simulink model "Electrical_System_2018b_obfs"  (R2019b)
settings: Solver=VariableStepAuto  StartTime=0.0  StopTime=5  RelTol=1e-3  AbsTol=1e-3  EnableMultiTasking=on
InitFcn:
  | Steady_State_Initialisation;
StopFcn:
  | %sscexplore(simlog);
  | %Logging
undefined symbols (not defined in the file): abrlhklxvp, aexgmhuedq, afmfmjnutg, afpphrjpnc, ahuxbyvruc, alarvljztt, amxnyqmnuw, aodrlwvqie, aolhmuplyq, aqpmguuqkg, auesgwirzl, aurophlnng, awamelrhru, ayfhvxflxn, azxkacuhqc, babszerikg, bawhdqanwq, bevoqecvei, bltjvqbchx, bmqsuewujl, bsmyqjfgnf, btvjbsmnve, bywgxqeadw, bziaduxaer, bzmcmdqocb, bzsvyvetat, ccsjnrbsih, cdvenygxwh, cedkrnslhx, cjheorclzs, cjrdshrtqx, ckhavyhcza, ckxewznhlz, cmrcgyiplk, conenicnws, cqkejbgjnn, csfnuwymhe, cunupkhwbh, cwzfvzuxxh, dcadmadufn, dcfponivnv, ddtrqjrhjn, dfhoxvkqas, dfrhtcwpne, dfvomcagjv, djijwylxea, dnmeqksrrm, dnzewbdkaa, dsqcykyxav, dtswwlttmm, ecumpidjtv, edegaywrct, ejjjsmnejc, eknqnehjdz, emvdetzouf, esxbqkbahr, etnkkbreiq, eunoiiiirw, ewewcuedir, fatkfxdhtc ... (+386)
libraries: fl_lib x802, ee_lib x362, fl_ps_legacy_lib x160, nesl_utility x85
(part 12 of 26)

== system Electrical_System_2018b_obfs/Redacted_1221/Redacted_7996/Redacted_1/Redacted_4377/Redacted_6082/Redacted_6448 ==
  Redacted_2500 : ee_lib/Semiconductors & Converters/Diode  ModelType=efectnzfzk  Vf=jxmepmeowj V  Ron=qgxsnpyvap Ohm  Goff=yoppabgzkl S  prmExp=ubpcccmurz  I12=remshksgqe A  V12=lfyuowwnsp V  IS=kniawzssyt A  ec=shjfprvpho  I1=bqvkznozbx A  V1=kanhzjgbwy V  RS=xqskwtorcu Ohm  Tmeas=wkndwwjeju degC  N_series=oemgleyaog  N_parallel=rmwesacawc  Rz=uupgbnboph Ohm  BV=jmlshjudem V  C_param=ejznuqydbf  CJ=jnyvftnijl pF  CJ0=eocfcshsjc pF  VJ=rcqumjutus V  Mgrad=bpwyttzsav  Vvec=xmbkulzqwe V  Cvec=eqgbafiqja pF  FC=fzcbcscgmr  Q_param=hevnohlimn  iRM=fkisxhzojn A  iF=aecufenajy A  didt=wqayegsgya A/us  trr_factor=tyozkzrsye  trr=byygrqxzxs ns  Qrr=ecsprgxdxa s*uA  TT=estselsvjb ns  tau=lnvjuifvwe ns  T_param=jrnxklcvyp  IS_T2=pegzeyggnh A  I1_T2=dfmjfojaum A  V1_T2=dkkcmajvzi V  Tmeas2=mhkasfkmys degC  EG_param=agwssckltu  EG=rfaarmrbja eV  XTI_param=uxzupvrblg  XTI=ospysejegc  dBVdT=tootsfdmyr V/K  Tdevice=kzpnsiiwfr degC  i_specify=off  i_priority=None  i=eihvzvfrzd A  i_nominal_specify=off  i_nominal_unit=A  i_nominal_value=qmmhrurogd  v_specify=off  v_priority=None  v=hizlbruxfz V  v_nominal_specify=off  v_nominal_unit=V  v_nominal_value=ycpyizpqai  i_capacitor_specify=off  i_capacitor_priority=None  i_capacitor=zppifvcjba A  i_capacitor_nominal_specify=off  i_capacitor_nominal_unit=A  i_capacitor_nominal_value=fpmjfabdfd  v_capacitor_specify=off  v_capacitor_priority=None  v_capacitor=stollmyrll V  v_capacitor_nominal_specify=off  v_capacitor_nominal_unit=V  v_capacitor_nominal_value=kndonlhkoo  power_dissipated_specify=off  power_dissipated_priority=None  power_dissipated=btdavdcdiv W  power_dissipated_nominal_specify=off  power_dissipated_nominal_unit=W  power_dissipated_nominal_value=tkklgbzblp  thermal_network_parameterization=bljrklmcju  Rth=xhsqylwmob K/W  Rth_Foster=optpcutsoi K/W  thermal_mass_parameterization=ugcqtdtype  thermal_mass=jsyutsyost J/K  thermal_mass_Foster=twrmylwkjc J/K  thermal_time_constant=xnykkposzd s  thermal_time_constant_Foster=foiqukjmop s  thermal_mass_initial_temperatures=upiyseqegs degC
      settings: SourceProductName=Simscape Electrical  InternalSimscapePortConfiguration="{\"Bottom\":[],\"Left\":[{\"id\":\"p\",\"label\":\"\",\"type\":\"foundation.electrical.electrical\"},{\"id\":\"H\",\"label\":\"H\",\"type\":\"foundation.thermal.thermal\"}],\"Right\":[{\"id\":\"n\",\"label\":\"\",\"type\":\"foundation.electrical.electrical\"}],\"Top\":[]}"
  Redacted_359 : ee_lib/Semiconductors & Converters/Diode  ModelType=scvaiquffk  Vf=gurupglfta V  Ron=ftlaqddzvo Ohm  Goff=sbgfdffxay S  prmExp=ukcnmjtiae  I12=grbxogokac A  V12=wmzyrlvpsn V  IS=leyegtjcol A  ec=lwvjfwcdkf  I1=dljtokvayx A  V1=irawojoicp V  RS=axoqkcbxfn Ohm  Tmeas=aargryzkwo degC  N_series=kaksezvljy  N_parallel=xdnjyjftou  Rz=rcunxliptk Ohm  BV=hrrjansjso V  C_param=gklskhmoru  CJ=imyuobqtwk pF  CJ0=ewdqrpecjy pF  VJ=wfjksexohd V  Mgrad=jgqtcmmwqv  Vvec=aguvzvrglj V  Cvec=zssvjevjde pF  FC=oeclxcixjt  Q_param=xrpxrrdafl  iRM=bcqzohazjt A  iF=crytmcfhbt A  didt=sirllclhmt A/us  trr_factor=ziidcweruu  trr=wxebnnxvyt ns  Qrr=ausdiytbgo s*uA  TT=naewcxqzgl ns  tau=ctbkxtppav ns  T_param=kyxkskcyft  IS_T2=nshgzahsri A  I1_T2=xuvyuqjsme A  V1_T2=oltorpmvrx V  Tmeas2=gktjbxgqtx degC  EG_param=iwktfixgrg  EG=teimjuixxi eV  XTI_param=shpugjdkdk  XTI=yrdjcsecbk  dBVdT=volhbyrkkf V/K  Tdevice=ofrafibacf degC  i_specify=off  i_priority=None  i=qtezljymoi A  i_nominal_specify=off  i_nominal_unit=A  i_nominal_value=yxnhkqaqti  v_specify=off  v_priority=None  v=kbwxruyprv V  v_nominal_specify=off  v_nominal_unit=V  v_nominal_value=igljubvsuu  i_capacitor_specify=off  i_capacitor_priority=None  i_capacitor=mlyqgxdfvw A  i_capacitor_nominal_specify=off  i_capacitor_nominal_unit=A  i_capacitor_nominal_value=ujbiigzksz  v_capacitor_specify=off  v_capacitor_priority=None  v_capacitor=cojyhmmzxj V  v_capacitor_nominal_specify=off  v_capacitor_nominal_unit=V  v_capacitor_nominal_value=wujzjvntdo  power_dissipated_specify=off  power_dissipated_priority=None  power_dissipated=yxytktehoc W  power_dissipated_nominal_specify=off  power_dissipated_nominal_unit=W  power_dissipated_nominal_value=pjafufeysq  thermal_network_parameterization=tftjmfuyfl  Rth=qburaojkwt K/W  Rth_Foster=jtrsywfksp K/W  thermal_mass_parameterization=mpaelmbuic  thermal_mass=qbntcmqzdf J/K  thermal_mass_Foster=iddtfueyvm J/K  thermal_time_constant=ewlbqfzhqf s  thermal_time_constant_Foster=ircpsmtrsx s  thermal_mass_initial_temperatures=xmifunpacs degC
      settings: SourceProductName=Simscape Electrical  InternalSimscapePortConfiguration="{\"Bottom\":[],\"Left\":[{\"id\":\"p\",\"label\":\"\",\"type\":\"foundation.electrical.electrical\"},{\"id\":\"H\",\"label\":\"H\",\"type\":\"foundation.thermal.thermal\"}],\"Right\":[{\"id\":\"n\",\"label\":\"\",\"type\":\"foundation.electrical.electrical\"}],\"Top\":[]}"
  Redacted_4119 : fl_lib/Electrical/Electrical Elements/Switch  R_closed=nvzhbxdgzi Ohm  G_open=jocuywfdlu 1/Ohm  Threshold=ycxpvyjhxx  i_specify=off  i_priority=None  i=wyjfxhkfvg A  i_nominal_specify=off  i_nominal_unit=A  i_nominal_value=qhiybsolgq  v_specify=off  v_priority=None  v=qhliplaqbe V  v_nominal_specify=off  v_nominal_unit=V  v_nominal_value=dflzoctfhv
      settings: SourceProductName=Simscape
  Redacted_7045 : ee_lib/Passive/Thermal/Thermal Resistor  R=znufdvpgrp K/W  T_specify=off  T_priority=None  T=gjhwzpgvuf K  T_nominal_specify=off  T_nominal_unit=K  T_nominal_value=wamkuaqotp  Q_specify=off  Q_priority=None  Q=iffnecxdnj W  Q_nominal_specify=off  Q_nominal_unit=W  Q_nominal_value=vfrfuelbtd
      settings: SourceProductName=Simscape Electrical  SourceProductBaseCode=PS  InternalSimscapePortConfiguration="{\"Bottom\":[],\"Left\":[{\"id\":\"A\",\"label\":\"A\",\"type\":\"foundation.thermal.thermal\"}],\"Right\":[{\"id\":\"B\",\"label\":\"B\",\"type\":\"foundation.thermal.thermal\"}],\"Top\":[]}"
  Redacted_7113 : fl_lib/Electrical/Electrical Elements/Switch  R_closed=xpgttbnlcv Ohm  G_open=qgroafvezw 1/Ohm  Threshold=emvdetzouf  i_specify=off  i_priority=None  i=kqcxlhjixi A  i_nominal_specify=off  i_nominal_unit=A  i_nominal_value=serpbanljy  v_specify=off  v_priority=None  v=tquhywvxiq V  v_nominal_specify=off  v_nominal_unit=V  v_nominal_value=hqozyjemvy
      settings: SourceProductName=Simscape
  Redacted_7754 : ee_lib/Passive/Thermal/Thermal Resistor  R=pifghqliop K/W  T_specify=off  T_priority=None  T=liaimvkskv K  T_nominal_specify=off  T_nominal_unit=K  T_nominal_value=plbwxvjplh  Q_specify=off  Q_priority=None  Q=nitcggggrk W  Q_nominal_specify=off  Q_nominal_unit=W  Q_nominal_value=cufaoxszsm
      settings: SourceProductName=Simscape Electrical  SourceProductBaseCode=PS  InternalSimscapePortConfiguration="{\"Bottom\":[],\"Left\":[{\"id\":\"A\",\"label\":\"A\",\"type\":\"foundation.thermal.thermal\"}],\"Right\":[{\"id\":\"B\",\"label\":\"B\",\"type\":\"foundation.thermal.thermal\"}],\"Top\":[]}"
  Redacted_8069 : ee_lib/Passive/Thermal/Thermal Resistor  R=ykpjzexeck K/W  T_specify=off  T_priority=None  T=dcfponivnv K  T_nominal_specify=off  T_nominal_unit=K  T_nominal_value=qfeaychhrh  Q_specify=off  Q_priority=None  Q=umsrugkwnq W  Q_nominal_specify=off  Q_nominal_unit=W  Q_nominal_value=pcplguatyr
      settings: SourceProductName=Simscape Electrical  SourceProductBaseCode=PS  InternalSimscapePortConfiguration="{\"Bottom\":[],\"Left\":[{\"id\":\"A\",\"label\":\"A\",\"type\":\"foundation.thermal.thermal\"}],\"Right\":[{\"id\":\"B\",\"label\":\"B\",\"type\":\"foundation.thermal.thermal\"}],\"Top\":[]}"
  Redacted_9919 : PMIOPort  Side=Left
  Redacted_9600 : PMIOPort  Port=2  Side=Left
  Redacted_2456 : PMIOPort  Port=3  Side=Right
  Redacted_124 : PMIOPort  Port=4  Side=Right
  Redacted_8053 : PMIOPort  Port=5  Side=Left
  Redacted_4129 : PMIOPort  Port=6  Side=Right
  connections:
  Redacted_2500/LConn1 -- Redacted_9600/RConn1
  Redacted_2500/RConn1 -- Redacted_7113/LConn1
  Redacted_359/LConn2 -- Redacted_8069/LConn1
  Redacted_2456/RConn1 -- Redacted_4119/RConn2
  Redacted_359/LConn1 -- Redacted_4119/LConn1
  Redacted_9919/RConn1 -- Redacted_359/RConn1
  Redacted_7754/RConn1 -- Redacted_7045/LConn1 -- Redacted_8069/RConn1
  Redacted_4129/RConn1 -- Redacted_7113/RConn1 -- Redacted_4119/RConn1
  Redacted_124/RConn1 -- Redacted_7113/RConn2
  Redacted_7045/RConn1 -- Redacted_8053/RConn1
  Redacted_2500/LConn2 -- Redacted_7754/LConn1

== system Electrical_System_2018b_obfs/Redacted_1221/Redacted_7996/Redacted_1/Redacted_4377/Redacted_6082/Redacted_6527 ==
  Redacted_1424 : fl_lib/Electrical/Electrical Elements/Switch  R_closed=uubemsahiq Ohm  G_open=ozvememgqv 1/Ohm  Threshold=hnjmvnuswb  i_specify=off  i_priority=None  i=itzyracony A  i_nominal_specify=off  i_nominal_unit=A  i_nominal_value=zqxgqfenru  v_specify=off  v_priority=None  v=wleqakrbwd V  v_nominal_specify=off  v_nominal_unit=V  v_nominal_value=wygbutdclo
      settings: SourceProductName=Simscape
  Redacted_1733 : ee_lib/Passive/Thermal/Thermal Resistor  R=qgzigcwvwq K/W  T_specify=off  T_priority=None  T=vssqyrasqs K  T_nominal_specify=off  T_nominal_unit=K  T_nominal_value=uvmszgxxre  Q_specify=off  Q_priority=None  Q=jpywnaxojq W  Q_nominal_specify=off  Q_nominal_unit=W  Q_nominal_value=kkwfnufnoo
      settings: SourceProductName=Simscape Electrical  SourceProductBaseCode=PS  InternalSimscapePortConfiguration="{\"Bottom\":[],\"Left\":[{\"id\":\"A\",\"label\":\"A\",\"type\":\"foundation.thermal.thermal\"}],\"Right\":[{\"id\":\"B\",\"label\":\"B\",\"type\":\"foundation.thermal.thermal\"}],\"Top\":[]}"
  Redacted_2307 : ee_lib/Semiconductors & Converters/Diode  ModelType=yygispdsap  Vf=ddgocjgltc V  Ron=fwvfaxzvnp Ohm  Goff=wfblsuugok S  prmExp=qxzndhluss  I12=sqshvrdiph A  V12=nfodczazgj V  IS=whobbihuku A  ec=abzzdvvrza  I1=rdkvkqhdyd A  V1=zvbmipings V  RS=jpbkbpprev Ohm  Tmeas=nwhqotdbur degC  N_series=tfmhjxhjrz  N_parallel=begksghsae  Rz=ruutgskgma Ohm  BV=knynobbzgk V  C_param=zzrudhbdpf  CJ=thqgethmmh pF  CJ0=bhxhuuybgj pF  VJ=wampydxduu V  Mgrad=eqjkzbyofp  Vvec=mmgcagzjpe V  Cvec=zawyetnrxx pF  FC=ahrrwotxui  Q_param=xzjdgflsym  iRM=agdsnvjalq A  iF=ffnfwdscvn A  didt=fdxjshyvxs A/us  trr_factor=mkmyfvfyes  trr=gacgpnqvgu ns  Qrr=bbyyevepig s*uA  TT=tucnxfnpvo ns  tau=jahxnwizgh ns  T_param=hcisegfjcv  IS_T2=cgermndsgq A  I1_T2=vpzanteidy A  V1_T2=ztiovvpyyv V  Tmeas2=wwduknfans degC  EG_param=nvxjhmwpig  EG=xogzvypibl eV  XTI_param=oyofysglfl  XTI=ktkazczzev  dBVdT=nymuoqofpc V/K  Tdevice=ytwxdnehpn degC  i_specify=off  i_priority=None  i=zbhtayrmow A  i_nominal_specify=off  i_nominal_unit=A  i_nominal_value=vbxoxffqhl  v_specify=off  v_priority=None  v=vksdaxyjuv V  v_nominal_specify=off  v_nominal_unit=V  v_nominal_value=kanmrfdloo  i_capacitor_specify=off  i_capacitor_priority=None  i_capacitor=axztnhmdly A  i_capacitor_nominal_specify=off  i_capacitor_nominal_unit=A  i_capacitor_nominal_value=zvchdgraoo  v_capacitor_specify=off  v_capacitor_priority=None  v_capacitor=pkrddeylhy V  v_capacitor_nominal_specify=off  v_capacitor_nominal_unit=V  v_capacitor_nominal_value=rrafgiklmt  power_dissipated_specify=off  power_dissipated_priority=None  power_dissipated=lxbrmovrpy W  power_dissipated_nominal_specify=off  power_dissipated_nominal_unit=W  power_dissipated_nominal_value=kpwlhtkzah  thermal_network_parameterization=ersljgwkre  Rth=dpxszekbmk K/W  Rth_Foster=sedshturqg K/W  thermal_mass_parameterization=hiobflsxct  thermal_mass=nanxcpyyrc J/K  thermal_mass_Foster=swbqkjbtue J/K  thermal_time_constant=ogdijojbab s  thermal_time_constant_Foster=poxzlosyls s  thermal_mass_initial_temperatures=vuabxoysws degC
      settings: SourceProductName=Simscape Electrical  InternalSimscapePortConfiguration="{\"Bottom\":[],\"Left\":[{\"id\":\"p\",\"label\":\"\",\"type\":\"foundation.electrical.electrical\"},{\"id\":\"H\",\"label\":\"H\",\"type\":\"foundation.thermal.thermal\"}],\"Right\":[{\"id\":\"n\",\"label\":\"\",\"type\":\"foundation.electrical.electrical\"}],\"Top\":[]}"
  Redacted_5471 : ee_lib/Semiconductors & Converters/Diode  ModelType=dylqyfrumb  Vf=djwjlavxgg V  Ron=wjabrhhflf Ohm  Goff=ozauqfzfha S  prmExp=ieadlxwboq  I12=vpknywidyi A  V12=kxgzcqifbg V  IS=vcjqsyxitp A  ec=xvocbgesta  I1=huqetrpfgu A  V1=iynwjgmjhg V  RS=epzvhgmnsg Ohm  Tmeas=xqcholenhs degC  N_series=akurbozukz  N_parallel=lpafsotiku  Rz=dksbfwxken Ohm  BV=fowtsskggn V  C_param=mnpnfxxqye  CJ=aicgqixsbh pF  CJ0=srulofhfse pF  VJ=ouozluioet V  Mgrad=gfwibmsyze  Vvec=zaumleognr V  Cvec=yumfhvbkfs pF  FC=oqewfcqqju  Q_param=dsbrgeddbn  iRM=oaxjisldwr A  iF=swkfaahtjk A  didt=lebtvikjdv A/us  trr_factor=aswjjjyqva  trr=lhjvtwshym ns  Qrr=juuqdlouyy s*uA  TT=hpxbjdimvz ns  tau=ejuitcqjpx ns  T_param=vtnictwnru  IS_T2=bwporktges A  I1_T2=epinzvdzxw A  V1_T2=vcakwitolb V  Tmeas2=ufhgbygray degC  EG_param=beqjzgrucc  EG=ysoejqncmm eV  XTI_param=ybyrlmockc  XTI=dftuoysnwu  dBVdT=nefgclzwgj V/K  Tdevice=mljvtbjnva degC  i_specify=off  i_priority=None  i=jwadwmquns A  i_nominal_specify=off  i_nominal_unit=A  i_nominal_value=gktrqjynpb  v_specify=off  v_priority=None  v=njcctfkoay V  v_nominal_specify=off  v_nominal_unit=V  v_nominal_value=jxheyghequ  i_capacitor_specify=off  i_capacitor_priority=None  i_capacitor=vmzfsoqwwu A  i_capacitor_nominal_specify=off  i_capacitor_nominal_unit=A  i_capacitor_nominal_value=qrccizfisq  v_capacitor_specify=off  v_capacitor_priority=None  v_capacitor=cxinpvqodn V  v_capacitor_nominal_specify=off  v_capacitor_nominal_unit=V  v_capacitor_nominal_value=apzgnesosv  power_dissipated_specify=off  power_dissipated_priority=None  power_dissipated=hgheroluap W  power_dissipated_nominal_specify=off  power_dissipated_nominal_unit=W  power_dissipated_nominal_value=phjvibdzdg  thermal_network_parameterization=givzvrzuan  Rth=iixviegddv K/W  Rth_Foster=gsdmkgpcqm K/W  thermal_mass_parameterization=zqrrqkoaxz  thermal_mass=fvqhopbxbu J/K  thermal_mass_Foster=hysvxqdxyw J/K  thermal_time_constant=yatkhnfcgl s  thermal_time_constant_Foster=ojtticlvlv s  thermal_mass_initial_temperatures=bmufljunea degC
      settings: SourceProductName=Simscape Electrical  InternalSimscapePortConfiguration="{\"Bottom\":[],\"Left\":[{\"id\":\"p\",\"label\":\"\",\"type\":\"foundation.electrical.electrical\"},{\"id\":\"H\",\"label\":\"H\",\"type\":\"foundation.thermal.thermal\"}],\"Right\":[{\"id\":\"n\",\"label\":\"\",\"type\":\"foundation.electrical.electrical\"}],\"Top\":[]}"
  Redacted_5989 : ee_lib/Passive/Thermal/Thermal Resistor  R=ytpfqnyozy K/W  T_specify=off  T_priority=None  T=rfkrxpivtt K  T_nominal_specify=off  T_nominal_unit=K  T_nominal_value=dvmqgiitak  Q_specify=off  Q_priority=None  Q=npjdipshuc W  Q_nominal_specify=off  Q_nominal_unit=W  Q_nominal_value=eerlcjerke
      settings: SourceProductName=Simscape Electrical  SourceProductBaseCode=PS  InternalSimscapePortConfiguration="{\"Bottom\":[],\"Left\":[{\"id\":\"A\",\"label\":\"A\",\"type\":\"foundation.thermal.thermal\"}],\"Right\":[{\"id\":\"B\",\"label\":\"B\",\"type\":\"foundation.thermal.thermal\"}],\"Top\":[]}"
  Redacted_6325 : fl_lib/Electrical/Electrical Elements/Switch  R_closed=arlniknull Ohm  G_open=hcbdoqshtz 1/Ohm  Threshold=qqftcuuewi  i_specify=off  i_priority=None  i=mltdghhuuz A  i_nominal_specify=off  i_nominal_unit=A  i_nominal_value=tzrqlrltkl  v_specify=off  v_priority=None  v=edsdzxsadv V  v_nominal_specify=off  v_nominal_unit=V  v_nominal_value=niuolmioqy
      settings: SourceProductName=Simscape
  Redacted_9115 : ee_lib/Passive/Thermal/Thermal Resistor  R=vruipktyzb K/W  T_specify=off  T_priority=None  T=qsufbscrtd K  T_nominal_specify=off  T_nominal_unit=K  T_nominal_value=grbzvqfklm  Q_specify=off  Q_priority=None  Q=htwqzangcg W  Q_nominal_specify=off  Q_nominal_unit=W  Q_nominal_value=uchgmkqgfm
      settings: SourceProductName=Simscape Electrical  SourceProductBaseCode=PS  InternalSimscapePortConfiguration="{\"Bottom\":[],\"Left\":[{\"id\":\"A\",\"label\":\"A\",\"type\":\"foundation.thermal.thermal\"}],\"Right\":[{\"id\":\"B\",\"label\":\"B\",\"type\":\"foundation.thermal.thermal\"}],\"Top\":[]}"
  Redacted_6828 : PMIOPort  Side=Left
  Redacted_6214 : PMIOPort  Port=2  Side=Left
  Redacted_7583 : PMIOPort  Port=3  Side=Right
  Redacted_3746 : PMIOPort  Port=4  Side=Right
  Redacted_1539 : PMIOPort  Port=5  Side=Left
  Redacted_7195 : PMIOPort  Port=6  Side=Right
  connections:
  Redacted_5471/LConn2 -- Redacted_5989/LConn1
  Redacted_1733/RConn1 -- Redacted_1539/RConn1
  Redacted_3746/RConn1 -- Redacted_6325/RConn2
  Redacted_1424/RConn1 -- Redacted_6325/RConn1 -- Redacted_7195/RConn1
  Redacted_9115/RConn1 -- Redacted_1733/LConn1 -- Redacted_5989/RConn1
  Redacted_6828/RConn1 -- Redacted_2307/RConn1
  Redacted_2307/LConn1 -- Redacted_1424/LConn1
  Redacted_7583/RConn1 -- Redacted_1424/RConn2
  Redacted_2307/LConn2 -- Redacted_9115/LConn1
  Redacted_5471/RConn1 -- Redacted_6325/LConn1
  Redacted_5471/LConn1 -- Redacted_6214/RConn1

== system Electrical_System_2018b_obfs/Redacted_1221/Redacted_7996/Redacted_1/Redacted_4377/Redacted_6082/Redacted_6620 ==
  Redacted_2014 : ee_lib/Semiconductors & Converters/Diode  ModelType=gqiqleufpp  Vf=rciegaahyr V  Ron=izpyebfwtu Ohm  Goff=knahxehrum S  prmExp=gfxklcgmfk  I12=sbznuevzft A  V12=qpwzodqtgo V  IS=ebxfpmarae A  ec=cwkebwdiwj  I1=hqlohoyszw A  V1=mibkackcep V  RS=jhziukqmxk Ohm  Tmeas=tipcupyvvg degC  N_series=agpfoieknu  N_parallel=pauhaoalka  Rz=zxlwwxndwh Ohm  BV=swupfoviat V  C_param=ttoktqetan  CJ=mfxdwlmbvb pF  CJ0=ffeyzckaxr pF  VJ=nuecpjtket V  Mgrad=zfikmwifnf  Vvec=phbjpfbebd V  Cvec=jhnyxymlxo pF  FC=qfmmxpjbpo  Q_param=tjqqjjtelq  iRM=zutwrbrukx A  iF=pfiaynnkdw A  didt=zeupzzuvaz A/us  trr_factor=xhypptopno  trr=jkwajzgcje ns  Qrr=wowpcqfxws s*uA  TT=ypsxdlnldi ns  tau=nitvzeaztq ns  T_param=swaejwrfsv  IS_T2=xjhdogbuoa A  I1_T2=ldlggurlak A  V1_T2=obdohodlqe V  Tmeas2=tbryjoyfon degC  EG_param=erphnnwltu  EG=brjowwryvb eV  XTI_param=owdxpyfvwu  XTI=hgcqikgdha  dBVdT=lrzjaamqpw V/K  Tdevice=tcrbomkdjd degC  i_specify=off  i_priority=None  i=hqtjudspyd A  i_nominal_specify=off  i_nominal_unit=A  i_nominal_value=bwqxfkinvz  v_specify=off  v_priority=None  v=hjzmmprpyc V  v_nominal_specify=off  v_nominal_unit=V  v_nominal_value=njncclngsw  i_capacitor_specify=off  i_capacitor_priority=None  i_capacitor=ciyrjytfew A  i_capacitor_nominal_specify=off  i_capacitor_nominal_unit=A  i_capacitor_nominal_value=siexlgmunl  v_capacitor_specify=off  v_capacitor_priority=None  v_capacitor=xpshqsgilj V  v_capacitor_nominal_specify=off  v_capacitor_nominal_unit=V  v_capacitor_nominal_value=hpsiplsygj  power_dissipated_specify=off  power_dissipated_priority=None  power_dissipated=juqfttnpie W  power_dissipated_nominal_specify=off  power_dissipated_nominal_unit=W  power_dissipated_nominal_value=lyxbmpxuee  thermal_network_parameterization=ysuejmoxwn  Rth=finvmqpapu K/W  Rth_Foster=qosqwhtwdn K/W  thermal_mass_parameterization=swzmoavdkp  thermal_mass=ywjpsxqlmn J/K  thermal_mass_Foster=zzqhnpotok J/K  thermal_time_constant=ifknfrcsyy s  thermal_time_constant_Foster=pykgbenxxp s  thermal_mass_initial_temperatures=kgoranomvt degC
      settings: SourceProductName=Simscape Electrical  InternalSimscapePortConfiguration="{\"Bottom\":[],\"Left\":[{\"id\":\"p\",\"label\":\"\",\"type\":\"foundation.electrical.electrical\"},{\"id\":\"H\",\"label\":\"H\",\"type\":\"foundation.thermal.thermal\"}],\"Right\":[{\"id\":\"n\",\"label\":\"\",\"type\":\"foundation.electrical.electrical\"}],\"Top\":[]}"
  Redacted_2373 : fl_lib/Electrical/Electrical Elements/Switch  R_closed=kdyjcggfxg Ohm  G_open=afvdermyno 1/Ohm  Threshold=tjabhhlnxp  i_specify=off  i_priority=None  i=qurnjndsab A  i_nominal_specify=off  i_nominal_unit=A  i_nominal_value=znixxagswj  v_specify=off  v_priority=None  v=xqjhhmdgoi V  v_nominal_specify=off  v_nominal_unit=V  v_nominal_value=bwgubpgymn
      settings: SourceProductName=Simscape
  Redacted_328 : ee_lib/Passive/Thermal/Thermal Resistor  R=kxydmktclb K/W  T_specify=off  T_priority=None  T=vxwjbstjgr K  T_nominal_specify=off  T_nominal_unit=K  T_nominal_value=seidpjimmz  Q_specify=off  Q_priority=None  Q=ywgtndhhrq W  Q_nominal_specify=off  Q_nominal_unit=W  Q_nominal_value=kiultrtaba
      settings: SourceProductName=Simscape Electrical  SourceProductBaseCode=PS  InternalSimscapePortConfiguration="{\"Bottom\":[],\"Left\":[{\"id\":\"A\",\"label\":\"A\",\"type\":\"foundation.thermal.thermal\"}],\"Right\":[{\"id\":\"B\",\"label\":\"B\",\"type\":\"foundation.thermal.thermal\"}],\"Top\":[]}"
  Redacted_5690 : ee_lib/Passive/Thermal/Thermal Resistor  R=jddwcmhgli K/W  T_specify=off  T_priority=None  T=zezvrnfoms K  T_nominal_specify=off  T_nominal_unit=K  T_nominal_value=mzautmapaq  Q_specify=off  Q_priority=None  Q=yyadonrfbk W  Q_nominal_specify=off  Q_nominal_unit=W  Q_nominal_value=uclyfxddyt
      settings: SourceProductName=Simscape Electrical  SourceProductBaseCode=PS  InternalSimscapePortConfiguration="{\"Bottom\":[],\"Left\":[{\"id\":\"A\",\"label\":\"A\",\"type\":\"foundation.thermal.thermal\"}],\"Right\":[{\"id\":\"B\",\"label\":\"B\",\"type\":\"foundation.thermal.thermal\"}],\"Top\":[]}"
  Redacted_5845 : fl_lib/Electrical/Electrical Elements/Switch  R_closed=icjvxdmcka Ohm  G_open=kexskzpskw 1/Ohm  Threshold=ckhavyhcza  i_specify=off  i_priority=None  i=ahqiwrglzv A  i_nominal_specify=off  i_nominal_unit=A  i_nominal_value=mqjcwkekap  v_specify=off  v_priority=None  v=nvxykueeox V  v_nominal_specify=off  v_nominal_unit=V  v_nominal_value=ndecikrhmu
      settings: SourceProductName=Simscape
  Redacted_7283 : ee_lib/Semiconductors & Converters/Diode  ModelType=rzispxqwda  Vf=gnrpcrdaiq V  Ron=ghfqfgqnjp Ohm  Goff=ymfjoafqzi S  prmExp=tqesvxwkea  I12=gozxalvtjw A  V12=pfyubiyuoh V  IS=mbclrzefme A  ec=okvrwbwosn  I1=jpahbfupht A  V1=vpjuinocqb V  RS=brkyhzgmwm Ohm  Tmeas=zpdstripvt degC  N_series=stuuhiyehn  N_parallel=trqngxgybj  Rz=nzotohhllu Ohm  BV=opywdvhnir V  C_param=yuoevnzdrc  CJ=dhacxrqtkw pF  CJ0=mcyeruteos pF  VJ=mcmizpovly V  Mgrad=vsutktjlwr  Vvec=xuzjzmvewr V  Cvec=chlneajmrc pF  FC=nlhhtnylay  Q_param=cehpwvemhb  iRM=rlczpfgyem A  iF=ksurhnqwmp A  didt=idojsdbupn A/us  trr_factor=vejvrsmbmm  trr=kgmamwjxvx ns  Qrr=sefksjtwpk s*uA  TT=ifvfcwpbar ns  tau=mktlcufgsp ns  T_param=oprpphkwsn  IS_T2=ojtnhwzapa A  I1_T2=otxdgcfkfq A  V1_T2=fvsufutiqn V  Tmeas2=wipgwptrgf degC  EG_param=jbkevzjnlz  EG=ygoaixicyx eV  XTI_param=lgjkmxsxep  XTI=quhynflpcu  dBVdT=zwfbrmsbta V/K  Tdevice=phqcsvszoj degC  i_specify=off  i_priority=None  i=gjjcexnudv A  i_nominal_specify=off  i_nominal_unit=A  i_nominal_value=cfpddevnes  v_specify=off  v_priority=None  v=euxehncunu V  v_nominal_specify=off  v_nominal_unit=V  v_nominal_value=lplxzeyrex  i_capacitor_specify=off  i_capacitor_priority=None  i_capacitor=tbylysbvet A  i_capacitor_nominal_specify=off  i_capacitor_nominal_unit=A  i_capacitor_nominal_value=klnsswlrcx  v_capacitor_specify=off  v_capacitor_priority=None  v_capacitor=sxnwccbswb V  v_capacitor_nominal_specify=off  v_capacitor_nominal_unit=V  v_capacitor_nominal_value=yowydohudj  power_dissipated_specify=off  power_dissipated_priority=None  power_dissipated=cgphorjmje W  power_dissipated_nominal_specify=off  power_dissipated_nominal_unit=W  power_dissipated_nominal_value=fvywpxahim  thermal_network_parameterization=tyffilnlux  Rth=skkjpribxf K/W  Rth_Foster=hnqwerdzfk K/W  thermal_mass_parameterization=vwchogqojn  thermal_mass=xrttmmxuwx J/K  thermal_mass_Foster=oxwxslpupn J/K  thermal_time_constant=mxcjwvzono s  thermal_time_constant_Foster=gwwbtvmuug s  thermal_mass_initial_temperatures=claqdpboor degC
      settings: SourceProductName=Simscape Electrical  InternalSimscapePortConfiguration="{\"Bottom\":[],\"Left\":[{\"id\":\"p\",\"label\":\"\",\"type\":\"foundation.electrical.electrical\"},{\"id\":\"H\",\"label\":\"H\",\"type\":\"foundation.thermal.thermal\"}],\"Right\":[{\"id\":\"n\",\"label\":\"\",\"type\":\"foundation.electrical.electrical\"}],\"Top\":[]}"
  Redacted_9450 : ee_lib/Passive/Thermal/Thermal Resistor  R=wlxdrklwxe K/W  T_specify=off  T_priority=None  T=ncdbkbrldr K  T_nominal_specify=off  T_nominal_unit=K  T_nominal_value=tpldjyjupo  Q_specify=off  Q_priority=None  Q=wtqakfmuxk W  Q_nominal_specify=off  Q_nominal_unit=W  Q_nominal_value=wvihfdufoh
      settings: SourceProductName=Simscape Electrical  SourceProductBaseCode=PS  InternalSimscapePortConfiguration="{\"Bottom\":[],\"Left\":[{\"id\":\"A\",\"label\":\"A\",\"type\":\"foundation.thermal.thermal\"}],\"Right\":[{\"id\":\"B\",\"label\":\"B\",\"type\":\"foundation.thermal.thermal\"}],\"Top\":[]}"
  Redacted_4655 : PMIOPort  Side=Left
  Redacted_6502 : PMIOPort  Port=2  Side=Left
  Redacted_6154 : PMIOPort  Port=3  Side=Right
  Redacted_874 : PMIOPort  Port=4  Side=Right
  Redacted_3696 : PMIOPort  Port=5  Side=Left
  Redacted_2870 : PMIOPort  Port=6  Side=Right
  connections:
  Redacted_7283/LConn1 -- Redacted_6502/RConn1
  Redacted_7283/RConn1 -- Redacted_5845/LConn1
  Redacted_2014/LConn2 -- Redacted_9450/LConn1
  Redacted_6154/RConn1 -- Redacted_2373/RConn2
  Redacted_2014/LConn1 -- Redacted_2373/LConn1
  Redacted_4655/RConn1 -- Redacted_2014/RConn1
  Redacted_5690/RConn1 -- Redacted_328/LConn1 -- Redacted_9450/RConn1
  Redacted_2870/RConn1 -- Redacted_5845/RConn1 -- Redacted_2373/RConn1
  Redacted_874/RConn1 -- Redacted_5845/RConn2
  Redacted_328/RConn1 -- Redacted_3696/RConn1
  Redacted_7283/LConn2 -- Redacted_5690/LConn1

== system Electrical_System_2018b_obfs/Redacted_1221/Redacted_7996/Redacted_1/Redacted_4377/Redacted_6082/Redacted_6805 ==
  Redacted_3337 : fl_lib/Electrical/Electrical Elements/Switch  R_closed=yxjpulldun Ohm  G_open=kegtkujuqm 1/Ohm  Threshold=liaknalfrc  i_specify=off  i_priority=None  i=vfyyawjcai A  i_nominal_specify=off  i_nominal_unit=A  i_nominal_value=qcjaunzuqi  v_specify=off  v_priority=None  v=swbfgzjayv V  v_nominal_specify=off  v_nominal_unit=V  v_nominal_value=ccklftegqq
      settings: SourceProductName=Simscape
  Redacted_4658 : ee_lib/Passive/Thermal/Thermal Resistor  R=cjheorclzs K/W  T_specify=off  T_priority=None  T=oxllrndvxl K  T_nominal_specify=off  T_nominal_unit=K  T_nominal_value=vttfcznyjj  Q_specify=off  Q_priority=None  Q=veltrvmbzh W  Q_nominal_specify=off  Q_nominal_unit=W  Q_nominal_value=iyxxiklgjl
      settings: SourceProductName=Simscape Electrical  SourceProductBaseCode=PS  InternalSimscapePortConfiguration="{\"Bottom\":[],\"Left\":[{\"id\":\"A\",\"label\":\"A\",\"type\":\"foundation.thermal.thermal\"}],\"Right\":[{\"id\":\"B\",\"label\":\"B\",\"type\":\"foundation.thermal.thermal\"}],\"Top\":[]}"
  Redacted_4994 : ee_lib/Passive/Thermal/Thermal Resistor  R=gypqteikkp K/W  T_specify=off  T_priority=None  T=oshyvpbftq K  T_nominal_specify=off  T_nominal_unit=K  T_nominal_value=ncwvhuakjs  Q_specify=off  Q_priority=None  Q=vojlmgegxo W  Q_nominal_specify=off  Q_nominal_unit=W  Q_nominal_value=fvyiuwsylh
      settings: SourceProductName=Simscape Electrical  SourceProductBaseCode=PS  InternalSimscapePortConfiguration="{\"Bottom\":[],\"Left\":[{\"id\":\"A\",\"label\":\"A\",\"type\":\"foundation.thermal.thermal\"}],\"Right\":[{\"id\":\"B\",\"label\":\"B\",\"type\":\"foundation.thermal.thermal\"}],\"Top\":[]}"
  Redacted_585 : fl_lib/Electrical/Electrical Elements/Switch  R_closed=wdigxdpfas Ohm  G_open=lafhprgygd 1/Ohm  Threshold=aolhmuplyq  i_specify=off  i_priority=None  i=vcdeejycwc A  i_nominal_specify=off  i_nominal_unit=A  i_nominal_value=ershxznodz  v_specify=off  v_priority=None  v=irimjohetc V  v_nominal_specify=off  v_nominal_unit=V  v_nominal_value=bejlrppchs
      settings: SourceProductName=Simscape
  Redacted_7139 : ee_lib/Passive/Thermal/Thermal Resistor  R=qokdevsgjk K/W  T_specify=off  T_priority=None  T=zzfqycdapp K  T_nominal_specify=off  T_nominal_unit=K  T_nominal_value=mlevfhnhhd  Q_specify=off  Q_priority=None  Q=grrzcklvos W  Q_nominal_specify=off  Q_nominal_unit=W  Q_nominal_value=pjoujutyxi
      settings: SourceProductName=Simscape Electrical  SourceProductBaseCode=PS  InternalSimscapePortConfiguration="{\"Bottom\":[],\"Left\":[{\"id\":\"A\",\"label\":\"A\",\"type\":\"foundation.thermal.thermal\"}],\"Right\":[{\"id\":\"B\",\"label\":\"B\",\"type\":\"foundation.thermal.thermal\"}],\"Top\":[]}"
  Redacted_7477 : ee_lib/Semiconductors & Converters/Diode  ModelType=siopqsdkke  Vf=vlytbuckhg V  Ron=dnkirfiwtb Ohm  Goff=hybfzeduao S  prmExp=kwsebrwvgd  I12=kfsmyoqzna A  V12=hnkonhxsbr V  IS=isykihjzmv A  ec=yrzkujitpm  I1=dhfqeyhuyd A  V1=zgsewcozym V  RS=mpcljitwmr Ohm  Tmeas=ebrkobcskh degC  N_series=cblbppjhmu  N_parallel=gcijoxluxf  Rz=wwudmfsgii Ohm  BV=ywubfrqvzl V  C_param=ufueahyemx  CJ=ucffunbhjr pF  CJ0=gvgqkuhnif pF  VJ=eafaphsqye V  Mgrad=stbyrblvuf  Vvec=lqtyuphlxe V  Cvec=kwepiurgav pF  FC=bocziebzeh  Q_param=axqhxumszd  iRM=mvlaklwalt A  iF=fvdwflwmxq A  didt=yduxgmzydl A/us  trr_factor=xzyzzmdibz  trr=mqeokcuxni ns  Qrr=eacuvomyfz s*uA  TT=wqeovxwgoy ns  tau=icgjzejdcm ns  T_param=qvfyrqpkio  IS_T2=tyrvatdotb A  I1_T2=hdybxwnxgg A  V1_T2=ocskkzbdfs V  Tmeas2=roeazaidao degC  EG_param=ltrdisotaf  EG=irbxnhvhnf eV  XTI_param=uvozxekhry  XTI=vcneuywdti  dBVdT=bjxifjvwqu V/K  Tdevice=lzvjtpnwvt degC  i_specify=off  i_priority=None  i=yyxgeutxkj A  i_nominal_specify=off  i_nominal_unit=A  i_nominal_value=hkglitcqqq  v_specify=off  v_priority=None  v=ncxmzzrzjk V  v_nominal_specify=off  v_nominal_unit=V  v_nominal_value=lsdkgzvlcc  i_capacitor_specify=off  i_capacitor_priority=None  i_capacitor=xlhxuygwjg A  i_capacitor_nominal_specify=off  i_capacitor_nominal_unit=A  i_capacitor_nominal_value=drafximium  v_capacitor_specify=off  v_capacitor_priority=None  v_capacitor=jpwbpwcwee V  v_capacitor_nominal_specify=off  v_capacitor_nominal_unit=V  v_capacitor_nominal_value=hdkefavzlf  power_dissipated_specify=off  power_dissipated_priority=None  power_dissipated=sarhttkwql W  power_dissipated_nominal_specify=off  power_dissipated_nominal_unit=W  power_dissipated_nominal_value=mavrwpomwo  thermal_network_parameterization=lrcygnfvyi  Rth=srgsdzcvpf K/W  Rth_Foster=twreyxnsjr K/W  thermal_mass_parameterization=nbdhbesxpg  thermal_mass=rxfluekgwa J/K  thermal_mass_Foster=cklbgtlgis J/K  thermal_time_constant=lubwmajmlm s  thermal_time_constant_Foster=tnksfxwvyl s  thermal_mass_initial_temperatures=cgflfnvnmx degC
      settings: SourceProductName=Simscape Electrical  InternalSimscapePortConfiguration="{\"Bottom\":[],\"Left\":[{\"id\":\"p\",\"label\":\"\",\"type\":\"foundation.electrical.electrical\"},{\"id\":\"H\",\"label\":\"H\",\"type\":\"foundation.thermal.thermal\"}],\"Right\":[{\"id\":\"n\",\"label\":\"\",\"type\":\"foundation.electrical.electrical\"}],\"Top\":[]}"
  Redacted_7606 : ee_lib/Semiconductors & Converters/Diode  ModelType=uzkzrdmcdd  Vf=rmmzroxgij V  Ron=gmhtedufnv Ohm  Goff=jjlyzatkvo S  prmExp=veirngjlfx  I12=qvvduldzrp A  V12=zynirzrnpf V  IS=wxxxvpohgl A  ec=fplwtkcwyr  I1=kpelximtdu A  V1=wylxnblunc V  RS=jbawbkggmq Ohm  Tmeas=bayoigkdqj degC  N_series=bgulwrfglp  N_parallel=khxpeniani  Rz=lylxbzffke Ohm  BV=csvlicgnxf V  C_param=wxpimfnkor  CJ=rlhvodbzhe pF  CJ0=tjvrgdxdbq pF  VJ=kymohesfqq V  Mgrad=exkywwsvhl  Vvec=xkmmhtmqkw V  Cvec=fymvnufolq pF  FC=tgeertiozj  Q_param=yijflpurri  iRM=fjtqudaeyk A  iF=opauyjbtnw A  didt=wdwvlihuzw A/us  trr_factor=olttdrnnql  trr=egrhxizosf ns  Qrr=lsshsmphht s*uA  TT=edtwkkrcoh ns  tau=raidgjkdvk ns  T_param=ahbhdfhjai  IS_T2=ekcwzeqyaw A  I1_T2=orjhprekra A  V1_T2=ztliozxhxg V  Tmeas2=tfrmoaghps degC  EG_param=oapwdsvvtf  EG=irybcfpwlp eV  XTI_param=olnutyjuem  XTI=xesgdyozdg  dBVdT=oepeppyrik V/K  Tdevice=jpqttphnsz degC  i_specify=off  i_priority=None  i=svdtmokjoo A  i_nominal_specify=off  i_nominal_unit=A  i_nominal_value=abngkcnppn  v_specify=off  v_priority=None  v=uaenfqikhz V  v_nominal_specify=off  v_nominal_unit=V  v_nominal_value=ptrurkjdbb  i_capacitor_specify=off  i_capacitor_priority=None  i_capacitor=qrsrlqghol A  i_capacitor_nominal_specify=off  i_capacitor_nominal_unit=A  i_capacitor_nominal_value=ndtskdbzxd  v_capacitor_specify=off  v_capacitor_priority=None  v_capacitor=drqgaqzvul V  v_capacitor_nominal_specify=off  v_capacitor_nominal_unit=V  v_capacitor_nominal_value=ufwludarpz  power_dissipated_specify=off  power_dissipated_priority=None  power_dissipated=zarwoastjt W  power_dissipated_nominal_specify=off  power_dissipated_nominal_unit=W  power_dissipated_nominal_value=yqmounopok  thermal_network_parameterization=lbqkpegruw  Rth=wfrzaaeyrf K/W  Rth_Foster=orzhpmmvoh K/W  thermal_mass_parameterization=cvfxrzqybx  thermal_mass=vploeluiax J/K  thermal_mass_Foster=fxfiinqkbf J/K  thermal_time_constant=wfhctbbpau s  thermal_time_constant_Foster=nxdwubasmi s  thermal_mass_initial_temperatures=izxzueqzis degC
      settings: SourceProductName=Simscape Electrical  InternalSimscapePortConfiguration="{\"Bottom\":[],\"Left\":[{\"id\":\"p\",\"label\":\"\",\"type\":\"foundation.electrical.electrical\"},{\"id\":\"H\",\"label\":\"H\",\"type\":\"foundation.thermal.thermal\"}],\"Right\":[{\"id\":\"n\",\"label\":\"\",\"type\":\"foundation.electrical.electrical\"}],\"Top\":[]}"
  Redacted_2990 : PMIOPort  Side=Left
  Redacted_5799 : PMIOPort  Port=2  Side=Left
  Redacted_5060 : PMIOPort  Port=3  Side=Right
  Redacted_1541 : PMIOPort  Port=4  Side=Right
  Redacted_1201 : PMIOPort  Port=5  Side=Left
  Redacted_6993 : PMIOPort  Port=6  Side=Right
  connections:
  Redacted_7477/LConn1 -- Redacted_5799/RConn1
  Redacted_7477/RConn1 -- Redacted_3337/LConn1
  Redacted_7606/LConn2 -- Redacted_7139/LConn1
  Redacted_5060/RConn1 -- Redacted_585/RConn2
  Redacted_7606/LConn1 -- Redacted_585/LConn1
  Redacted_2990/RConn1 -- Redacted_7606/RConn1
  Redacted_4994/RConn1 -- Redacted_4658/LConn1 -- Redacted_7139/RConn1
  Redacted_6993/RConn1 -- Redacted_3337/RConn1 -- Redacted_585/RConn1
  Redacted_1541/RConn1 -- Redacted_3337/RConn2
  Redacted_4658/RConn1 -- Redacted_1201/RConn1
  Redacted_7477/LConn2 -- Redacted_4994/LConn1

== system Electrical_System_2018b_obfs/Redacted_1221/Redacted_7996/Redacted_1/Redacted_4377/Redacted_6082/Redacted_7051 ==
  Neutral_Negative : Subsystem  VariantControl=Variant1
  Positive_Neutral : Subsystem  VariantControl=Variant3
  Redacted_1021 : Subsystem  VariantControl=Variant2
  Redacted_2697 : PMIOPort  Side=Left
  Redacted_1518 : PMIOPort  Port=2  Side=Left
  Redacted_2395 : PMIOPort  Port=3  Side=Left
  Redacted_3537 : PMIOPort  Port=4  Side=Right
  Redacted_8383 : PMIOPort  Port=5  Side=Right

== system Electrical_System_2018b_obfs/Redacted_1221/Redacted_7996/Redacted_1/Redacted_4377/Redacted_6082/Redacted_7167 ==
  Redacted_1303 : ee_lib/Passive/Thermal/Thermal Resistor  R=zbwmizebwe K/W  T_specify=off  T_priority=None  T=rqecdygusj K  T_nominal_specify=off  T_nominal_unit=K  T_nominal_value=lamojxsfir  Q_specify=off  Q_priority=None  Q=dlcstliuma W  Q_nominal_specify=off  Q_nominal_unit=W  Q_nominal_value=tijbovpdks
      settings: SourceProductName=Simscape Electrical  SourceProductBaseCode=PS  InternalSimscapePortConfiguration="{\"Bottom\":[],\"Left\":[{\"id\":\"A\",\"label\":\"A\",\"type\":\"foundation.thermal.thermal\"}],\"Right\":[{\"id\":\"B\",\"label\":\"B\",\"type\":\"foundation.thermal.thermal\"}],\"Top\":[]}"
  Redacted_2941 : ee_lib/Passive/Thermal/Thermal Resistor  R=dfhoxvkqas K/W  T_specify=off  T_priority=None  T=jlvbuiuarv K  T_nominal_specify=off  T_nominal_unit=K  T_nominal_value=nfbcsilcng  Q_specify=off  Q_priority=None  Q=dpepytyjnn W  Q_nominal_specify=off  Q_nominal_unit=W  Q_nominal_value=eutxhekizl
      settings: SourceProductName=Simscape Electrical  SourceProductBaseCode=PS  InternalSimscapePortConfiguration="{\"Bottom\":[],\"Left\":[{\"id\":\"A\",\"label\":\"A\",\"type\":\"foundation.thermal.thermal\"}],\"Right\":[{\"id\":\"B\",\"label\":\"B\",\"type\":\"foundation.thermal.thermal\"}],\"Top\":[]}"
  Redacted_3917 : fl_lib/Electrical/Electrical Elements/Switch  R_closed=eomshdfjtq Ohm  G_open=eawwctyuef 1/Ohm  Threshold=nqsqjnzstw  i_specify=off  i_priority=None  i=gvnqmmhjic A  i_nominal_specify=off  i_nominal_unit=A  i_nominal_value=mwmoxwopsr  v_specify=off  v_priority=None  v=gqkvmmaeai V  v_nominal_specify=off  v_nominal_unit=V  v_nominal_value=euweqcpati
      settings: SourceProductName=Simscape
  Redacted_615 : ee_lib/Semiconductors & Converters/Diode  ModelType=pgkejxjdjs  Vf=xdcykktqir V  Ron=eayqiytylj Ohm  Goff=xzfhydetzu S  prmExp=tdufjhjcbn  I12=hparrpdjbc A  V12=zqwdfgidjk V  IS=pexhzonywb A  ec=mqktskfdqf  I1=tcyogdxzfi A  V1=baszszoezq V  RS=bxlpeeaqsl Ohm  Tmeas=tbiklxcmxf degC  N_series=eikuqooelh  N_parallel=xnclysjpwz  Rz=svpfhmlvnd Ohm  BV=ymvvdallkk V  C_param=auiedyngha  CJ=tdcyeazvtn pF  CJ0=yhsttyriji pF  VJ=oyfcsuwtca V  Mgrad=ssglilauuc  Vvec=tcaqzincyj V  Cvec=gaeocfhldf pF  FC=govhvunkzb  Q_param=gwouayihiu  iRM=gmuyhfsqfq A  iF=qgolhenzzh A  didt=roskpmqafp A/us  trr_factor=rgtcsetsdw  trr=evtippvdri ns  Qrr=asluyjhcqx s*uA  TT=hthltjmqxb ns  tau=mpvzluyvkf ns  T_param=ffjfzvgxwk  IS_T2=wfxjsgcogp A  I1_T2=lfwejdvrcx A  V1_T2=peppezqval V  Tmeas2=yreqhveqgb degC  EG_param=dqtocyjvqe  EG=aodkzgenxb eV  XTI_param=ncbiefewza  XTI=uvmuxgsyie  dBVdT=ejtxbvomre V/K  Tdevice=gpojnnavgh degC  i_specify=off  i_priority=None  i=ylnqkojcnb A  i_nominal_specify=off  i_nominal_unit=A  i_nominal_value=rmjbnjurkm  v_specify=off  v_priority=None  v=igzgyorjhh V  v_nominal_specify=off  v_nominal_unit=V  v_nominal_value=llpsdzaxev  i_capacitor_specify=off  i_capacitor_priority=None  i_capacitor=phioximztf A  i_capacitor_nominal_specify=off  i_capacitor_nominal_unit=A  i_capacitor_nominal_value=zpfkwwvufw  v_capacitor_specify=off  v_capacitor_priority=None  v_capacitor=orgrxnzlgw V  v_capacitor_nominal_specify=off  v_capacitor_nominal_unit=V  v_capacitor_nominal_value=kmrqvqymze  power_dissipated_specify=off  power_dissipated_priority=None  power_dissipated=tckulawdha W  power_dissipated_nominal_specify=off  power_dissipated_nominal_unit=W  power_dissipated_nominal_value=zqxclxuaeb  thermal_network_parameterization=xbiounqwbn  Rth=cthaouvkmz K/W  Rth_Foster=ujuovdsbwu K/W  thermal_mass_parameterization=yndypypslu  thermal_mass=yqwtrsfarw J/K  thermal_mass_Foster=uknzmftfxw J/K  thermal_time_constant=gadiboyzjf s  thermal_time_constant_Foster=oonjgnxbhv s  thermal_mass_initial_temperatures=dwinptcuvn degC
      settings: SourceProductName=Simscape Electrical  InternalSimscapePortConfiguration="{\"Bottom\":[],\"Left\":[{\"id\":\"p\",\"label\":\"\",\"type\":\"foundation.electrical.electrical\"},{\"id\":\"H\",\"label\":\"H\",\"type\":\"foundation.thermal.thermal\"}],\"Right\":[{\"id\":\"n\",\"label\":\"\",\"type\":\"foundation.electrical.electrical\"}],\"Top\":[]}"
  Redacted_6479 : fl_lib/Electrical/Electrical Elements/Switch  R_closed=pbrfqnpyma Ohm  G_open=cpoeuurqry 1/Ohm  Threshold=xzfpsnkrcq  i_specify=off  i_priority=None  i=svmhsuqoiq A  i_nominal_specify=off  i_nominal_unit=A  i_nominal_value=grkinioqrq  v_specify=off  v_priority=None  v=bfmdrrxebu V  v_nominal_specify=off  v_nominal_unit=V  v_nominal_value=tuetnympor
      settings: SourceProductName=Simscape
  Redacted_6758 : ee_lib/Passive/Thermal/Thermal Resistor  R=udvbnpfogk K/W  T_specify=off  T_priority=None  T=stamifxejg K  T_nominal_specify=off  T_nominal_unit=K  T_nominal_value=jpdxtgtapc  Q_specify=off  Q_priority=None  Q=ijcjukjuex W  Q_nominal_specify=off  Q_nominal_unit=W  Q_nominal_value=ruzflvabxw
      settings: SourceProductName=Simscape Electrical  SourceProductBaseCode=PS  InternalSimscapePortConfiguration="{\"Bottom\":[],\"Left\":[{\"id\":\"A\",\"label\":\"A\",\"type\":\"foundation.thermal.thermal\"}],\"Right\":[{\"id\":\"B\",\"label\":\"B\",\"type\":\"foundation.thermal.thermal\"}],\"Top\":[]}"
  Redacted_950 : ee_lib/Semiconductors & Converters/Diode  ModelType=jinkuwtpek  Vf=atuwmhjlss V  Ron=nznnxbdyxy Ohm  Goff=ihbvkszwml S  prmExp=mibtplliji  I12=iyuliuqmcx A  V12=klduiyaqij V  IS=ikslmrckpw A  ec=zngamoehie  I1=jmqjtcgqqy A  V1=qeujplmsly V  RS=prjefekpfj Ohm  Tmeas=xbblauhoxo degC  N_series=zriukxbglf  N_parallel=xywdgylyct  Rz=mlyrjcrutc Ohm  BV=azpesxbvkt V  C_param=iwaqnxrihq  CJ=efrhdiawni pF  CJ0=wggafursrp pF  VJ=kimodzupzz V  Mgrad=zqomfqqbkp  Vvec=nmespqdqtf V  Cvec=ptwbjcbecf pF  FC=rhpfuhhgyh  Q_param=irgquspdkp  iRM=juwqonlivh A  iF=ngzsvssqdj A  didt=qpzzvxqyny A/us  trr_factor=ytjldsqsba  trr=ynapedjysl ns  Qrr=cxbfwkibab s*uA  TT=qdlmrgrjbk ns  tau=gxbazwmswf ns  T_param=jeqpakxjhj  IS_T2=oyhthfujhz A  I1_T2=slwpnostwc A  V1_T2=ufjvlweifr V  Tmeas2=dmcyrgyzee degC  EG_param=txmgcwnshd  EG=awhwjuusqu eV  XTI_param=ciqcncwotj  XTI=sbuczetxrl  dBVdT=vvkuzgntho V/K  Tdevice=ayjozqrwzo degC  i_specify=off  i_priority=None  i=lfrhocvsab A  i_nominal_specify=off  i_nominal_unit=A  i_nominal_value=ltsgntbaxv  v_specify=off  v_priority=None  v=etlymrjkwh V  v_nominal_specify=off  v_nominal_unit=V  v_nominal_value=epreckwkhm  i_capacitor_specify=off  i_capacitor_priority=None  i_capacitor=tmlxdjnhjw A  i_capacitor_nominal_specify=off  i_capacitor_nominal_unit=A  i_capacitor_nominal_value=qqxajawsrd  v_capacitor_specify=off  v_capacitor_priority=None  v_capacitor=upkznbdmiq V  v_capacitor_nominal_specify=off  v_capacitor_nominal_unit=V  v_capacitor_nominal_value=dtybisinlb  power_dissipated_specify=off  power_dissipated_priority=None  power_dissipated=hsiyqtyqwk W  power_dissipated_nominal_specify=off  power_dissipated_nominal_unit=W  power_dissipated_nominal_value=warucurcbx  thermal_network_parameterization=fzipsrgnag  Rth=uxblvsvlml K/W  Rth_Foster=lcjkmpdgtw K/W  thermal_mass_parameterization=pcvahjrfam  thermal_mass=cugzbrnibs J/K  thermal_mass_Foster=sinoggzltj J/K  thermal_time_constant=afzkjcdnxg s  thermal_time_constant_Foster=ypnpugavcs s  thermal_mass_initial_temperatures=kinrukpyro degC
      settings: SourceProductName=Simscape Electrical  InternalSimscapePortConfiguration="{\"Bottom\":[],\"Left\":[{\"id\":\"p\",\"label\":\"\",\"type\":\"foundation.electrical.electrical\"},{\"id\":\"H\",\"label\":\"H\",\"type\":\"foundation.thermal.thermal\"}],\"Right\":[{\"id\":\"n\",\"label\":\"\",\"type\":\"foundation.electrical.electrical\"}],\"Top\":[]}"
  Redacted_4250 : PMIOPort  Side=Left
  Redacted_3366 : PMIOPort  Port=2  Side=Left
  Redacted_6205 : PMIOPort  Port=3  Side=Right
  Redacted_8107 : PMIOPort  Port=4  Side=Right
  Redacted_7175 : PMIOPort  Port=5  Side=Left
  Redacted_7678 : PMIOPort  Port=6  Side=Right
  connections:
  Redacted_615/LConn1 -- Redacted_3366/RConn1
  Redacted_615/RConn1 -- Redacted_6479/LConn1
  Redacted_950/LConn2 -- Redacted_2941/LConn1
  Redacted_6205/RConn1 -- Redacted_3917/RConn2
  Redacted_950/LConn1 -- Redacted_3917/LConn1
  Redacted_4250/RConn1 -- Redacted_950/RConn1
  Redacted_6758/RConn1 -- Redacted_1303/LConn1 -- Redacted_2941/RConn1
  Redacted_7678/RConn1 -- Redacted_6479/RConn1 -- Redacted_3917/RConn1
  Redacted_8107/RConn1 -- Redacted_6479/RConn2
  Redacted_1303/RConn1 -- Redacted_7175/RConn1
  Redacted_615/LConn2 -- Redacted_6758/LConn1
